simulink model "MinSegShield_Demo_M1V3"  (R2013a)
settings: Solver=FixedStepDiscrete  SolverMode=SingleTasking  StartTime=0.0  StopTime=inf  FixedStep=.1  RelTol=1e-3
libraries: arduinolib x6
settings Model: SimulationMode=external  ExtModeTrigDuration=2  Creator=Alec  LastModifiedBy=hurstj
settings OptimizationCC: ExpressionDepthLimit=2147483647  OptimizeModelRefInitCode=on  LifeSpan=1
settings DebuggingCC: SolverPrmCheckMsg=none  StrictBusMsg=Warning
settings HardwareCC: ProdBitPerInt=16  ProdBitPerPointer=8  ProdIntDivRoundTo=Zero  ProdEndianess=LittleEndian  ProdWordSize=8  ProdHWDeviceType=Atmel->AVR
settings RTWCC: SystemTargetFile=realtime.tlc  GenerateMakefile=off  TemplateMakefile=realtime.tmf  Description=Real-Time Toolbox  RTWVerbose=off  ProcessScript=realtime_make_rtw_hook
settings CodeAppCC: CustomSymbolStrType=$N$R$M  InternalIdentifier=Classic
settings STFCustomTargetCC: TargetLibSuffix=.a  GenerateSampleERTMain=on  ERTCustomFileBanners=on  SupportNonInlinedSFcns=off  SupportVariableSizeSignals=on  MATLABClassNameForMDSCustomization=Simulink.SoftwareTarget.ERTCustomization  SystemTargetFile=realtime.tlc
settings ERTTargetCC: ParMdlRefBuildCompliant=off  CompOptLevelCompliant=off  ConcurrentExecutionCompliant=off  CombineOutputUpdateFcns=off  ERTFirstTimeCompliant=off  SupportContinuousTime=on  SupportVariableSizeSignals=on  ModelStepFunctionPrototypeControlCompliant=off  CPPClassGenCompliant=off  ExtMode=on  ExtModeTransport=3  ExtModeMexFile=ext_serial_win32_comm  ExtModeMexArgs=0 14 115200  ERTSrcFileBannerTemplate=realtime_code_template.cgt  ERTHdrFileBannerTemplate=realtime_code_template.cgt  ERTDataSrcFileTemplate=realtime_code_template.cgt  ERTDataHdrFileTemplate=realtime_code_template.cgt  ERTCustomFileTemplate=realtime_file_process.tlc

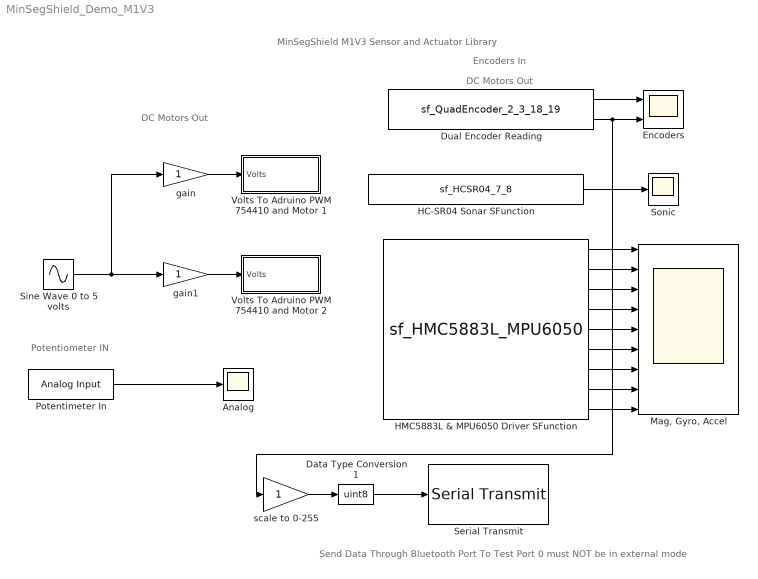
== system MinSegShield_Demo_M1V3 ==
  note: Send Data Through Bluetooth Port
      | To Test Port 0 must NOT be in external mode
  note: Potentiometer IN
  note: DC Motors Out
  note: DC Motors Out
  note: Encoders In
  note: MinSegShield M1V3 Sensor and Actuator Library
  Analog : Scope
      settings: TimeRange=30  YMin=200  YMax=1100  SaveName=ScopeData6
  Data Type Conversion1 : DataTypeConversion  OutDataTypeStr=uint8
  Dual Encoder Reading : S-Function  InitFcn=try, set_param(gcb,'FunctionName','sf_QuadEncoder_2_3_18_19'), end  FunctionName=sf_QuadEncoder_2_3_18_19  Parameters=uint8([0 1]),uint8([2 18]),uint8([3 19])  SFunctionModules=sf_QuadEncoder_2_3_18_19_wrapper  EnableBusSupport=off  mask(S-Function Builder){}
      mask init:
      | val = [[.9  0.75 0.75 1 1 .9 .9 1]',[1 1 0.75 0.75 .9 .9 1 .9]'];try , sys = get_param(gcb,'SfunBuilderFcnName');if isempty(sys), sys = get_param(gcb,'FunctionName'); end,catch, sys = get_param(gcb,'FunctionName'); end
      settings: CopyFcn=set_param(gcbh,'LinkStatus','none')  PreSaveFcn=try, set_param(gcb,'FunctionName','sf_QuadEncoder_2_3_18_19'), end  OpenFcn=sfunctionwizard(gcbh)
      mask Display: plot(val(:,1),val(:,2)),disp(sys), port_label('output',1,'pos1'), port_label('output',2,'pos2')
  Encoders : Scope  NumInputPorts=2
      settings: TimeRange=10  YMin=-700~-1  YMax=400~1
  HC-SR04 Sonar SFunction : S-Function  InitFcn=try, set_param(gcb,'FunctionName','sf_HCSR04_7_8'), end  FunctionName=sf_HCSR04_7_8  SFunctionModules=sf_HCSR04_7_8_wrapper  EnableBusSupport=off  mask(S-Function Builder){}
      mask help: Simulink:masks:SFunctionBuilder_MD
      mask init: same as MinSegShield_Demo_M1V3/Dual Encoder Reading
      settings: CopyFcn=set_param(gcbh,'LinkStatus','none')  PreSaveFcn=try, set_param(gcb,'FunctionName','sf_HCSR04_7_8'), end  OpenFcn=sfunctionwizard(gcbh)
      mask Display:
      | plot(val(:,1),val(:,2))
      | disp(sys)
      | port_label('output',1,'distance_cm')
  HMC5883L & MPU6050 Driver SFunction : S-Function  InitFcn=try, set_param(gcb,'FunctionName','sf_HMC5883L_MPU6050'), end  FunctionName=sf_HMC5883L_MPU6050  SFunctionModules=sf_HMC5883L_MPU6050_wrapper  EnableBusSupport=off  mask(S-Function Builder){}
      mask help: Simulink:masks:SFunctionBuilder_MD
      mask init: same as MinSegShield_Demo_M1V3/Dual Encoder Reading
      settings: CopyFcn=set_param(gcbh,'LinkStatus','none')  PreSaveFcn=try, set_param(gcb,'FunctionName','sf_HMC5883L_MPU6050'), end  OpenFcn=sfunctionwizard(gcbh)
      mask Display:
      | plot(val(:,1),val(:,2))
      | disp(sys)
      | port_label('output',1,'x_mag')
      | port_label('output',2,'y_mag')
      | port_label('output',3,'z_mag')
      | port_label('output',4,'x_vel')
      | port_label('output',5,'y_vel')
      | port_label('output',6,'z_vel')
      | port_label('output',7,'x_acc')
      | port_label('output',8,'y_acc')
      | port_label('output',9,'z_acc')
  "Mag, Gyro, Accel" : Scope  NumInputPorts=9
      settings: TimeRange=10  YMin=0~-300~-750~-15000~-2000~-20000~-7500~-7500~-5000  YMax=400~0~0~15000~1500~25000~7500~10000~20000
  Potentimeter In : arduinolib/Analog Input  pinNumber=0  sampleTime=-1
  Serial Transmit : arduinolib/Serial Transmit  portNumber=2
  Sine Wave 0 to 5 volts : Sin  SineType=Sample based  Amplitude=5  Frequency=50*2*pi  Samples=30  SampleTime=.1
  Sonic : Scope
      settings: TimeRange=30  YMin=0  YMax=175  SaveName=ScopeData2
  Volts To Adruino PWM 754410 and Motor 1 : Subsystem
  Volts To Adruino PWM 754410 and Motor 2 : Subsystem
  gain : Gain  OutDataTypeStr=int16
  gain1 : Gain  OutDataTypeStr=int16
  scale to 0-255 : Gain  OutDataTypeStr=int16
  wires:
  gain/1 -> Volts To Adruino PWM 754410 and Motor 1/1(Volts)
  Sine Wave 0 to 5 volts/1 -> gain1/1, gain/1
  gain1/1 -> Volts To Adruino PWM 754410 and Motor 2/1(Volts)
  Dual Encoder Reading/1 -> Encoders/1
  Dual Encoder Reading/2 -> scale to 0-255/1, Encoders/2
  HMC5883L & MPU6050 Driver SFunction/1 -> "Mag, Gyro, Accel"/1
  HMC5883L & MPU6050 Driver SFunction/2 -> "Mag, Gyro, Accel"/2
  HMC5883L & MPU6050 Driver SFunction/3 -> "Mag, Gyro, Accel"/3
  HMC5883L & MPU6050 Driver SFunction/4 -> "Mag, Gyro, Accel"/4
  HMC5883L & MPU6050 Driver SFunction/5 -> "Mag, Gyro, Accel"/5
  HMC5883L & MPU6050 Driver SFunction/6 -> "Mag, Gyro, Accel"/6
  HMC5883L & MPU6050 Driver SFunction/7 -> "Mag, Gyro, Accel"/7
  HMC5883L & MPU6050 Driver SFunction/8 -> "Mag, Gyro, Accel"/8
  HMC5883L & MPU6050 Driver SFunction/9 -> "Mag, Gyro, Accel"/9
  scale to 0-255/1 -> Data Type Conversion1/1
  Data Type Conversion1/1 -> Serial Transmit/1
  Potentimeter In/1 -> Analog/1
  HC-SR04 Sonar SFunction/1 -> Sonic/1

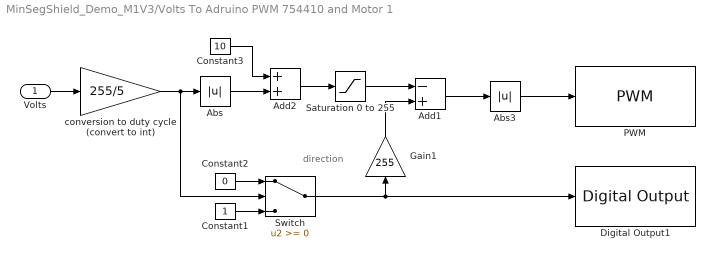
== system MinSegShield_Demo_M1V3/Volts To Adruino PWM 754410 and Motor 1 ==
  note: direction
  Volts : Inport
  Abs : Abs
  Abs3 : Abs
  Add1 : Sum  Inputs=-+
  Add2 : Sum
  Constant1 : Constant
  Constant2 : Constant  Value=0
  Constant3 : Constant  Value=10
  Digital Output1 : arduinolib/Digital Output  pinNumber=5
  Gain1 : Gain  Gain=255
  PWM : arduinolib/PWM  pinNumber=4
  Saturation 0 to 255 : Saturate  UpperLimit=255  LowerLimit=0
  Switch : Switch
  conversion to duty cycle (convert to int) : Gain  Gain=255/5  OutDataTypeStr=int16
  wires:
  Add2/1 -> Saturation 0 to 255/1
  Abs/1 -> Add2/2
  Constant3/1 -> Add2/1
  Abs3/1 -> PWM/1
  Saturation 0 to 255/1 -> Add1/1
  conversion to duty cycle (convert to int)/1 -> Abs/1, Switch/2
  Add1/1 -> Abs3/1
  Gain1/1 -> Add1/2
  Constant1/1 -> Switch/3
  Constant2/1 -> Switch/1
  Switch/1 -> Gain1/1, Digital Output1/1
  Volts/1 -> conversion to duty cycle (convert to int)/1

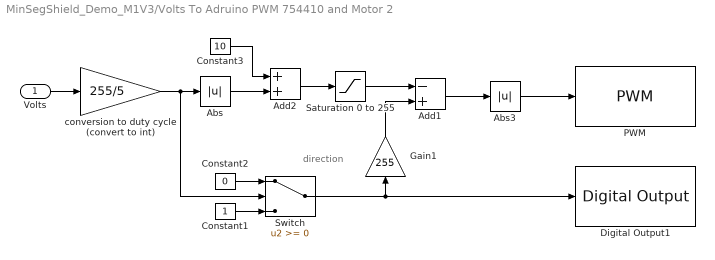
== system MinSegShield_Demo_M1V3/Volts To Adruino PWM 754410 and Motor 2 ==
  note: direction
  Volts : Inport
  Abs : Abs
  Abs3 : Abs
  Add1 : Sum  Inputs=-+
  Add2 : Sum
  Constant1 : Constant
  Constant2 : Constant  Value=0
  Constant3 : Constant  Value=10
  Digital Output1 : arduinolib/Digital Output  pinNumber=11
  Gain1 : Gain  Gain=255
  PWM : arduinolib/PWM  pinNumber=9
  Saturation 0 to 255 : Saturate  UpperLimit=255  LowerLimit=0
  Switch : Switch
  conversion to duty cycle (convert to int) : Gain  Gain=255/5  OutDataTypeStr=int16
  wires:
  Add2/1 -> Saturation 0 to 255/1
  Abs/1 -> Add2/2
  Constant3/1 -> Add2/1
  Abs3/1 -> PWM/1
  Saturation 0 to 255/1 -> Add1/1
  conversion to duty cycle (convert to int)/1 -> Abs/1, Switch/2
  Add1/1 -> Abs3/1
  Gain1/1 -> Add1/2
  Constant1/1 -> Switch/3
  Constant2/1 -> Switch/1
  Switch/1 -> Gain1/1, Digital Output1/1
  Volts/1 -> conversion to duty cycle (convert to int)/1
